simulink model "TEST_SensorSource_Lookup"  (R2020b)
settings: Solver=ode1  StartTime=tspan(1)  StopTime=tspan(2)  FixedStep=1/sensorFs.imuUpdateFs  RelTol=1e-3
values from neighbouring files (symbols this model uses):
  mag1 = double([Sensors.mag1.mag_x, Sensors.mag1.mag_y, Sensors.mag1.mag_z])    [navi_marg22.m]    (also in navi_marg24.m; navi_mvo17.m)
  mag2 = double([Sensors.mag2.mag_x, Sensors.mag2.mag_y, Sensors.mag2.mag_z])    [navi_marg22.m]    (also in navi_marg24.m; navi_mvo17.m)
  time = naviRes.time    [Plot_NaviMARG.m]    (also in UAVPlotLib.m = sensors.(sensorName).time; myplot_navfilter.m = sensors.Algo.time_algo; myplot_sensor_filter_compare.m = sensors.IMU.time_imu; postplot_marg_flightdata.m = sensors.Algo.time_algo)
undefined symbols (not defined in the file or in its folder): airspeed1, airspeed2, airspeed3, baro1, IMU1, IMU1_Control, IMU2, IMU3, laserDown1, laserDown2, radar1, radarLongDown1, radarLongForward1, sensorFs, ublox1, um482
(part 2 of 2)

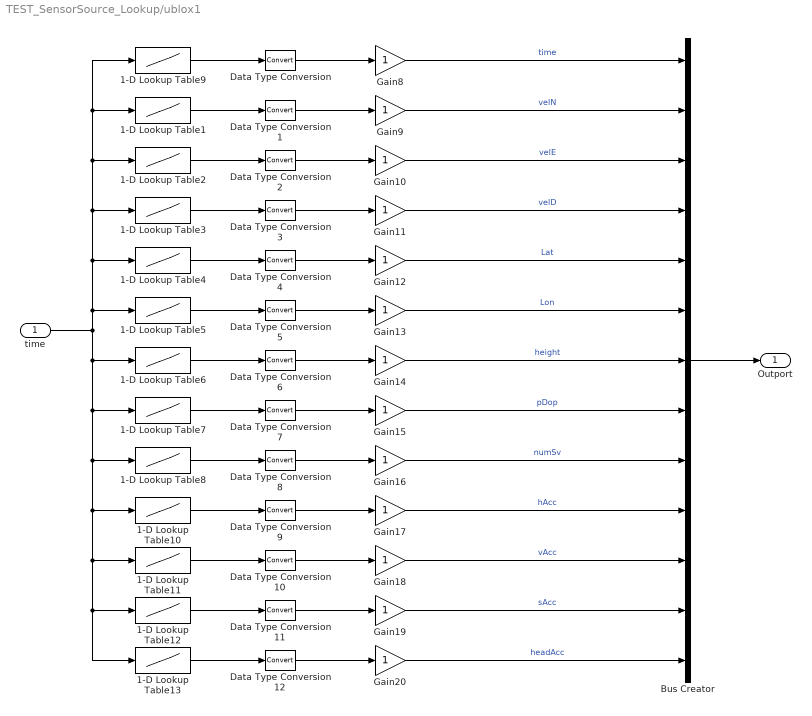
== system TEST_SensorSource_Lookup/ublox1 ==
  time : Inport
  1-D Lookup Table1 : Lookup_n-D  NumberOfTableDimensions=1  BreakpointsForDimension1=IN_SENSOR.ublox1.time(1:end-20)  Table=IN_SENSOR.ublox1.velN(1:end-20)  InterpMethod=Flat  ExtrapMethod=Clip  InternalRulePriority=Speed  RndMeth=Simplest  InputSameDT=on
  1-D Lookup Table10 : Lookup_n-D  NumberOfTableDimensions=1  BreakpointsForDimension1=IN_SENSOR.ublox1.time(1:end-20)  Table=IN_SENSOR.ublox1.hAcc(1:end-20)  InterpMethod=Flat  ExtrapMethod=Clip  InternalRulePriority=Speed  RndMeth=Simplest  InputSameDT=on
  1-D Lookup Table{9,11..13} (4 alike) : Lookup_n-D  NumberOfTableDimensions=1  BreakpointsForDimension1=IN_SENSOR.ublox1.time(1:end-20)  Table=IN_SENSOR.ublox1.time(1:end-20)  InterpMethod=Flat  ExtrapMethod=Clip  InternalRulePriority=Speed  RndMeth=Simplest  InputSameDT=on
  1-D Lookup Table2 : Lookup_n-D  NumberOfTableDimensions=1  BreakpointsForDimension1=IN_SENSOR.ublox1.time(1:end-20)  Table=IN_SENSOR.ublox1.velE(1:end-20)  InterpMethod=Flat  ExtrapMethod=Clip  InternalRulePriority=Speed  RndMeth=Simplest  InputSameDT=on
  1-D Lookup Table3 : Lookup_n-D  NumberOfTableDimensions=1  BreakpointsForDimension1=IN_SENSOR.ublox1.time(1:end-20)  Table=IN_SENSOR.ublox1.velD(1:end-20)  InterpMethod=Flat  ExtrapMethod=Clip  InternalRulePriority=Speed  RndMeth=Simplest  InputSameDT=on
  1-D Lookup Table4 : Lookup_n-D  NumberOfTableDimensions=1  BreakpointsForDimension1=IN_SENSOR.ublox1.time(1:end-20)  Table=IN_SENSOR.ublox1.Lat(1:end-20)  InterpMethod=Flat  ExtrapMethod=Clip  InternalRulePriority=Speed  RndMeth=Simplest  InputSameDT=on
  1-D Lookup Table5 : Lookup_n-D  NumberOfTableDimensions=1  BreakpointsForDimension1=IN_SENSOR.ublox1.time(1:end-20)  Table=IN_SENSOR.ublox1.Lon(1:end-20)  InterpMethod=Flat  ExtrapMethod=Clip  InternalRulePriority=Speed  RndMeth=Simplest  InputSameDT=on
  1-D Lookup Table6 : Lookup_n-D  NumberOfTableDimensions=1  BreakpointsForDimension1=IN_SENSOR.ublox1.time(1:end-20)  Table=IN_SENSOR.ublox1.height(1:end-20)  InterpMethod=Flat  ExtrapMethod=Clip  InternalRulePriority=Speed  RndMeth=Simplest  InputSameDT=on
  1-D Lookup Table7 : Lookup_n-D  NumberOfTableDimensions=1  BreakpointsForDimension1=IN_SENSOR.ublox1.time(1:end-20)  Table=IN_SENSOR.ublox1.pDop(1:end-20)  InterpMethod=Flat  ExtrapMethod=Clip  InternalRulePriority=Speed  RndMeth=Simplest  InputSameDT=on
  1-D Lookup Table8 : Lookup_n-D  NumberOfTableDimensions=1  BreakpointsForDimension1=IN_SENSOR.ublox1.time(1:end-20)  Table=IN_SENSOR.ublox1.numSv(1:end-20)  InterpMethod=Flat  ExtrapMethod=Clip  InternalRulePriority=Speed  RndMeth=Simplest  InputSameDT=on
  Bus Creator : BusCreator  Inputs=13
  Data Type Conversion{,1..12} (13 alike) : DataTypeConversion
  Gain{8..20} (13 alike) : Gain
  Outport : Outport
  wires:
  Gain16/1 -> Bus Creator/9  "numSv"
  Gain15/1 -> Bus Creator/8  "pDop"
  Gain14/1 -> Bus Creator/7  "height"
  Bus Creator/1 -> Outport/1
  Gain12/1 -> Bus Creator/5  "Lat"
  Gain8/1 -> Bus Creator/1  "time"
  Gain13/1 -> Bus Creator/6  "Lon"
  Gain9/1 -> Bus Creator/2  "velN"
  Gain10/1 -> Bus Creator/3  "velE"
  Gain11/1 -> Bus Creator/4  "velD"
  Gain17/1 -> Bus Creator/10  "hAcc"
  Gain18/1 -> Bus Creator/11  "vAcc"
  Gain19/1 -> Bus Creator/12  "sAcc"
  Gain20/1 -> Bus Creator/13  "headAcc"
  Data Type Conversion/1 -> Gain8/1
  1-D Lookup Table9/1 -> Data Type Conversion/1
  1-D Lookup Table1/1 -> Data Type Conversion1/1
  Data Type Conversion1/1 -> Gain9/1
  Data Type Conversion2/1 -> Gain10/1
  1-D Lookup Table2/1 -> Data Type Conversion2/1
  1-D Lookup Table3/1 -> Data Type Conversion3/1
  Data Type Conversion3/1 -> Gain11/1
  Data Type Conversion4/1 -> Gain12/1
  1-D Lookup Table4/1 -> Data Type Conversion4/1
  1-D Lookup Table5/1 -> Data Type Conversion5/1
  Data Type Conversion5/1 -> Gain13/1
  Data Type Conversion6/1 -> Gain14/1
  1-D Lookup Table6/1 -> Data Type Conversion6/1
  1-D Lookup Table7/1 -> Data Type Conversion7/1
  Data Type Conversion7/1 -> Gain15/1
  Data Type Conversion8/1 -> Gain16/1
  1-D Lookup Table8/1 -> Data Type Conversion8/1
  1-D Lookup Table10/1 -> Data Type Conversion9/1
  Data Type Conversion9/1 -> Gain17/1
  Data Type Conversion10/1 -> Gain18/1
  1-D Lookup Table11/1 -> Data Type Conversion10/1
  1-D Lookup Table12/1 -> Data Type Conversion11/1
  Data Type Conversion11/1 -> Gain19/1
  Data Type Conversion12/1 -> Gain20/1
  1-D Lookup Table13/1 -> Data Type Conversion12/1
  time/1 -> 1-D Lookup Table13/1, 1-D Lookup Table12/1, 1-D Lookup Table11/1, 1-D Lookup Table10/1, 1-D Lookup Table8/1, 1-D Lookup Table7/1, 1-D Lookup Table6/1, 1-D Lookup Table2/1, 1-D Lookup Table9/1, 1-D Lookup Table1/1, 1-D Lookup Table3/1, 1-D Lookup Table4/1, 1-D Lookup Table5/1

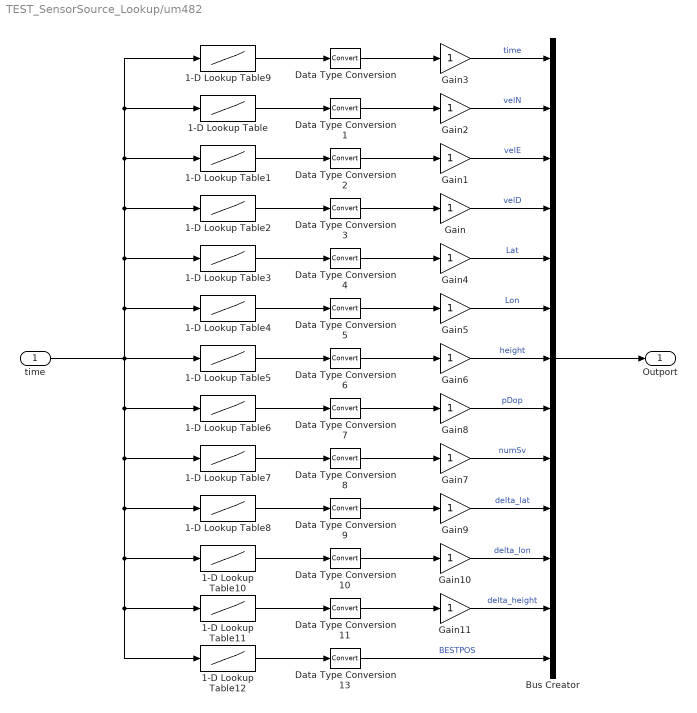
== system TEST_SensorSource_Lookup/um482 ==
  time : Inport
  1-D Lookup Table : Lookup_n-D  NumberOfTableDimensions=1  BreakpointsForDimension1=IN_SENSOR.um482.time(1:end-20)  Table=IN_SENSOR.um482.velN(1:end-20)  InterpMethod=Flat  ExtrapMethod=Clip  InternalRulePriority=Speed  RndMeth=Simplest  InputSameDT=on
  1-D Lookup Table1 : Lookup_n-D  NumberOfTableDimensions=1  BreakpointsForDimension1=IN_SENSOR.um482.time(1:end-20)  Table=IN_SENSOR.um482.velE(1:end-20)  InterpMethod=Flat  ExtrapMethod=Clip  InternalRulePriority=Speed  RndMeth=Simplest  InputSameDT=on
  1-D Lookup Table10 : Lookup_n-D  NumberOfTableDimensions=1  BreakpointsForDimension1=IN_SENSOR.um482.time(1:end-20)  Table=IN_SENSOR.um482.delta_lon(1:end-20)  InterpMethod=Flat  ExtrapMethod=Clip  InternalRulePriority=Speed  RndMeth=Simplest  InputSameDT=on
  1-D Lookup Table11 : Lookup_n-D  NumberOfTableDimensions=1  BreakpointsForDimension1=IN_SENSOR.um482.time(1:end-20)  Table=IN_SENSOR.um482.delta_height(1:end-20)  InterpMethod=Flat  ExtrapMethod=Clip  InternalRulePriority=Speed  RndMeth=Simplest  InputSameDT=on
  1-D Lookup Table12 : Lookup_n-D  NumberOfTableDimensions=1  BreakpointsForDimension1=IN_SENSOR.um482.time(1:end-20)  Table=IN_SENSOR.um482.BESTPOS(1:end-20)  InterpMethod=Flat  ExtrapMethod=Clip  InternalRulePriority=Speed  RndMeth=Simplest  InputSameDT=on
  1-D Lookup Table2 : Lookup_n-D  NumberOfTableDimensions=1  BreakpointsForDimension1=IN_SENSOR.um482.time(1:end-20)  Table=IN_SENSOR.um482.velD(1:end-20)  InterpMethod=Flat  ExtrapMethod=Clip  InternalRulePriority=Speed  RndMeth=Simplest  InputSameDT=on
  1-D Lookup Table3 : Lookup_n-D  NumberOfTableDimensions=1  BreakpointsForDimension1=IN_SENSOR.um482.time(1:end-20)  Table=IN_SENSOR.um482.Lat(1:end-20)  InterpMethod=Flat  ExtrapMethod=Clip  InternalRulePriority=Speed  RndMeth=Simplest  InputSameDT=on
  1-D Lookup Table4 : Lookup_n-D  NumberOfTableDimensions=1  BreakpointsForDimension1=IN_SENSOR.um482.time(1:end-20)  Table=IN_SENSOR.um482.Lon(1:end-20)  InterpMethod=Flat  ExtrapMethod=Clip  InternalRulePriority=Speed  RndMeth=Simplest  InputSameDT=on
  1-D Lookup Table5 : Lookup_n-D  NumberOfTableDimensions=1  BreakpointsForDimension1=IN_SENSOR.um482.time(1:end-20)  Table=IN_SENSOR.um482.height(1:end-20)  InterpMethod=Flat  ExtrapMethod=Clip  InternalRulePriority=Speed  RndMeth=Simplest  InputSameDT=on
  1-D Lookup Table6 : Lookup_n-D  NumberOfTableDimensions=1  BreakpointsForDimension1=IN_SENSOR.um482.time(1:end-20)  Table=IN_SENSOR.um482.pDop(1:end-20)  InterpMethod=Flat  ExtrapMethod=Clip  InternalRulePriority=Speed  RndMeth=Simplest  InputSameDT=on
  1-D Lookup Table7 : Lookup_n-D  NumberOfTableDimensions=1  BreakpointsForDimension1=IN_SENSOR.um482.time(1:end-20)  Table=IN_SENSOR.um482.numSv(1:end-20)  InterpMethod=Flat  ExtrapMethod=Clip  InternalRulePriority=Speed  RndMeth=Simplest  InputSameDT=on
  1-D Lookup Table8 : Lookup_n-D  NumberOfTableDimensions=1  BreakpointsForDimension1=IN_SENSOR.um482.time(1:end-20)  Table=IN_SENSOR.um482.delta_lat(1:end-20)  InterpMethod=Flat  ExtrapMethod=Clip  InternalRulePriority=Speed  RndMeth=Simplest  InputSameDT=on
  1-D Lookup Table9 : Lookup_n-D  NumberOfTableDimensions=1  BreakpointsForDimension1=IN_SENSOR.um482.time(1:end-20)  Table=IN_SENSOR.um482.time(1:end-20)  InterpMethod=Flat  ExtrapMethod=Clip  InternalRulePriority=Speed  RndMeth=Simplest  InputSameDT=on
  Bus Creator : BusCreator  Inputs=13
  Data Type Conversion{,1..11,13} (13 alike) : DataTypeConversion
  Gain{,1..11} (12 alike) : Gain
  Outport : Outport
  wires:
  Bus Creator/1 -> Outport/1
  Gain4/1 -> Bus Creator/5  "Lat"
  Gain6/1 -> Bus Creator/7  "height"
  Gain1/1 -> Bus Creator/3  "velE"
  Gain7/1 -> Bus Creator/9  "numSv"
  Gain/1 -> Bus Creator/4  "velD"
  Gain3/1 -> Bus Creator/1  "time"
  Gain2/1 -> Bus Creator/2  "velN"
  Gain5/1 -> Bus Creator/6  "Lon"
  Gain8/1 -> Bus Creator/8  "pDop"
  Gain9/1 -> Bus Creator/10  "delta_lat"
  Gain10/1 -> Bus Creator/11  "delta_lon"
  Gain11/1 -> Bus Creator/12  "delta_height"
  Data Type Conversion13/1 -> Bus Creator/13  "BESTPOS"
  time/1 -> 1-D Lookup Table11/1, 1-D Lookup Table12/1, 1-D Lookup Table10/1, 1-D Lookup Table8/1, 1-D Lookup Table7/1, 1-D Lookup Table6/1, 1-D Lookup Table9/1, 1-D Lookup Table/1, 1-D Lookup Table1/1, 1-D Lookup Table2/1, 1-D Lookup Table3/1, 1-D Lookup Table4/1, 1-D Lookup Table5/1
  1-D Lookup Table9/1 -> Data Type Conversion/1
  Data Type Conversion/1 -> Gain3/1
  Data Type Conversion1/1 -> Gain2/1
  1-D Lookup Table/1 -> Data Type Conversion1/1
  1-D Lookup Table2/1 -> Data Type Conversion3/1
  Data Type Conversion3/1 -> Gain/1
  Data Type Conversion2/1 -> Gain1/1
  1-D Lookup Table1/1 -> Data Type Conversion2/1
  1-D Lookup Table5/1 -> Data Type Conversion6/1
  Data Type Conversion6/1 -> Gain6/1
  Data Type Conversion7/1 -> Gain8/1
  1-D Lookup Table6/1 -> Data Type Conversion7/1
  1-D Lookup Table4/1 -> Data Type Conversion5/1
  Data Type Conversion5/1 -> Gain5/1
  Data Type Conversion4/1 -> Gain4/1
  1-D Lookup Table3/1 -> Data Type Conversion4/1
  1-D Lookup Table8/1 -> Data Type Conversion9/1
  Data Type Conversion9/1 -> Gain9/1
  Data Type Conversion10/1 -> Gain10/1
  1-D Lookup Table10/1 -> Data Type Conversion10/1
  1-D Lookup Table12/1 -> Data Type Conversion13/1
  Data Type Conversion11/1 -> Gain11/1
  1-D Lookup Table11/1 -> Data Type Conversion11/1
  Data Type Conversion8/1 -> Gain7/1
  1-D Lookup Table7/1 -> Data Type Conversion8/1
